simulink model "MSFartoystyring"  (R2017a)
settings: Solver=ode45  StartTime=tstart  StopTime=tstop  RelTol=1e-3  EnableMultiTasking=on
values from neighbouring files (symbols this model uses):
  c = 0    [run.m]    (also in run_task_2_2.m = 1; run_task_2_6.m = 1; run_task_2_6_without_crab_compensation.m = 1)
  chi_i_on = 0    [run_task_2_2.m]    (also in run_task_2_6.m = 1; run_task_2_6_without_crab_compensation.m)
  psi0 = 0    [run.m]    (also in run_task_2_2.m = 0.872664625997; run_task_2_6.m = 0.872664625997; run_task_2_6_without_crab_compensation.m = 0.872664625997)
  r0 = 0    [run.m]    (also in run_task_2_2.m; run_task_2_6.m; run_task_2_6_without_crab_compensation.m)
  tsamp = 10    [run.m]    (also in run_task_2_2.m; run_task_2_6.m; run_task_2_6_without_crab_compensation.m)
  v0 = [4.9 0]'    [run.m]    (also in run_task_2_2.m = [6.63 0]'; run_task_2_6.m = [6.63 0]'; run_task_2_6_without_crab_compensation.m = [6.63 0]')
undefined symbols (not defined in the file or in its folder): msfartoystyring, WP
undefined symbols (not defined in the file): p0
libraries: dspindex x2, dspswit3 x1
settings Model: ExtModeAutoUpdateStatusClock=off  Creator=christh  LastModifiedBy=jljoberg
settings DataIOCC: LimitDataPoints=on  SaveFormat=Array  SignalLoggingSaveFormat=ModelDataLogs
settings OptimizationCC: ExpressionDepthLimit=2147483647  InitFltsAndDblsToZero=on  LifeSpan=inf
settings DebuggingCC: UnderspecifiedInitializationDetection=Classic  MergeDetectMultiDrivingBlocksExec=none  SolverPrmCheckMsg=warning  StateNameClashWarn=warning  SFUnexpectedBacktrackingDiag=warning  SFNoUnconditionalDefaultTransitionDiag=warning  SFExecutionAtInitializationDiag=none
settings HardwareCC: ProdBitPerPointer=32  ProdBitPerSizeT=32  ProdBitPerPtrDiffT=32  ProdLargestAtomicFloat=None  ProdIntDivRoundTo=Undefined  ProdEndianess=Unspecified  ProdWordSize=32  ProdHWDeviceType=32-bit Generic
settings ModelReferenceCC: PropagateSignalLabelsOutOfModel=off
settings GRTTargetCC: TargetLangStandard=C89/C90 (ANSI)  GeneratePreprocessorConditionals=Disable all  CombineOutputUpdateFcns=off  GRTInterface=on
settings ConfigComp: CovMetricSettings=dw  CovHtmlReporting=on  CovSaveCumulativeToWorkspaceVar=on  CovSaveSingleToWorkspaceVar=on  CovExternalEMLEnable=off

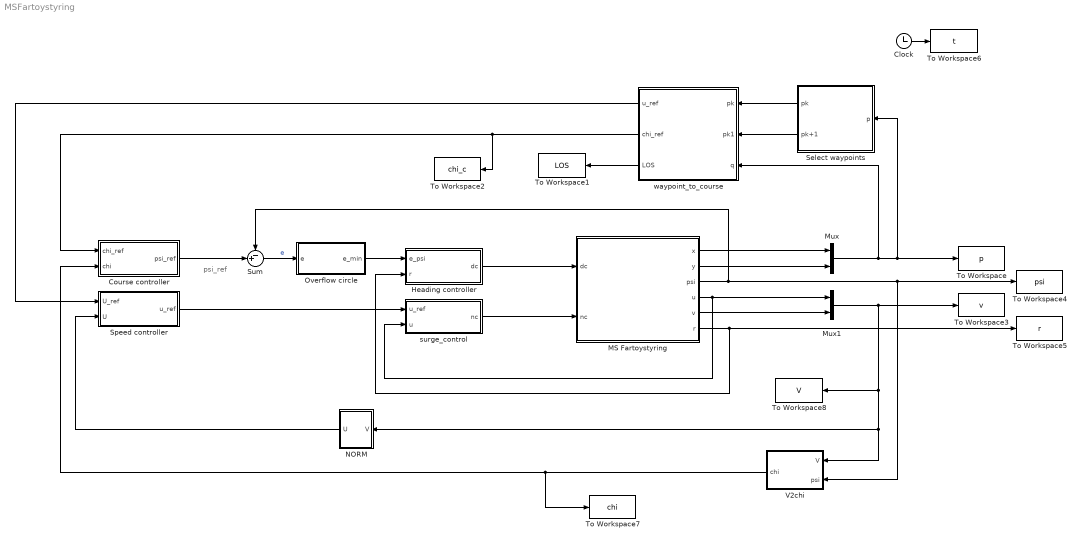
== system MSFartoystyring ==
  note: psi_ref
  Clock : Clock
  Course controller : Subsystem
  Heading controller : Subsystem
  MS Fartoystyring : Subsystem  mask(MS Fartoystyring for Assignment 3 G&C){x0=p0(1), y0=p0(2), u0=v0(1), v0=v0(2), psi0=psi0, r0=r0, c=c}
      mask prompts: x0 "x(t0) (m)"; y0 "y(t0) (m)"; u0 "u(t0) (m/s)"; v0 "v(t0) (m/s)"; psi0 "psi(t0) (rad)"; r0 "r(t0) (rad/s)"; c "current (0 or 1)"
      mask help:
      | Block corresponding to Figure 1 in the assignment text. Gives the response of the ship.
      |
      | The design speed of MS Fartoystyring is u=8.23 m/s.
      |
      | Input:
      | dc: commanded rudder (rad), dmax=25*pi/180
      | nc: commanded shaft speed (rad/s), nmax=85*2*pi/60
      |
      | Output:
      | x: north pos (m)
      | y: east pos (m)
      | u: surge (m/s)
      | v: sway (m/s)
      | psi: heading (rad)
      | r: yaw (rad/s)
      mask Help: Comments, bugs and help requests can be directed to the TA. Email on course website.
  Mux : Mux  Inputs=2
  Mux1 : Mux  Inputs=2
  NORM : MATLAB Function  TreatAsAtomicUnit=on
  Overflow circle : MATLAB Function  TreatAsAtomicUnit=on
  Select waypoints : Subsystem
  Speed controller : Subsystem
  Sum : Sum  Inputs=-+|
  To Workspace : ToWorkspace  VariableName=p  SampleTime=tsamp
  To Workspace1 : ToWorkspace  VariableName=LOS  SampleTime=tsamp
  To Workspace2 : ToWorkspace  VariableName=chi_c  SampleTime=tsamp
  To Workspace3 : ToWorkspace  VariableName=v  SampleTime=tsamp
  To Workspace4 : ToWorkspace  VariableName=psi  SampleTime=tsamp
  To Workspace5 : ToWorkspace  VariableName=r  SampleTime=tsamp
  To Workspace6 : ToWorkspace  VariableName=t  SampleTime=tsamp
  To Workspace7 : ToWorkspace  VariableName=chi  SampleTime=tsamp
  To Workspace8 : ToWorkspace  VariableName=V  SampleTime=tsamp
  V2chi : MATLAB Function  TreatAsAtomicUnit=on
  surge_control : Subsystem
  waypoint_to_course : MATLAB Function  TreatAsAtomicUnit=on
  wires:
  Clock/1 -> To Workspace6/1
  MS Fartoystyring/1(x) -> Mux/1
  MS Fartoystyring/2(y) -> Mux/2
  MS Fartoystyring/4(u) -> Mux1/1, surge_control/2(u)
  MS Fartoystyring/5(v) -> Mux1/2
  Mux1/1 -> To Workspace8/1, NORM/1(V), V2chi/1(V), To Workspace3/1
  MS Fartoystyring/6(r) -> Heading controller/2(r), To Workspace5/1
  waypoint_to_course/2(chi_ref) -> To Workspace2/1, Course controller/1(chi_ref)
  Select waypoints/1(pk) -> waypoint_to_course/1(pk)
  Select waypoints/2(pk+1) -> waypoint_to_course/2(pk1)
  Mux/1 -> To Workspace/1, Select waypoints/1(p), waypoint_to_course/3(q)
  waypoint_to_course/3(LOS) -> To Workspace1/1
  MS Fartoystyring/3(psi) -> Sum/1, To Workspace4/1, V2chi/2(psi)
  Sum/1 -> Overflow circle/1(e)  "e"
  Course controller/1(psi_ref) -> Sum/2
  surge_control/1(nc) -> MS Fartoystyring/2(nc)
  Overflow circle/1(e_min) -> Heading controller/1(e_psi)
  V2chi/1(chi) -> To Workspace7/1, Course controller/2(chi)
  Heading controller/1(dc) -> MS Fartoystyring/1(dc)
  waypoint_to_course/1(u_ref) -> Speed controller/1(U_ref)
  Speed controller/1(u_ref) -> surge_control/1(u_ref)
  NORM/1(U) -> Speed controller/2(U)

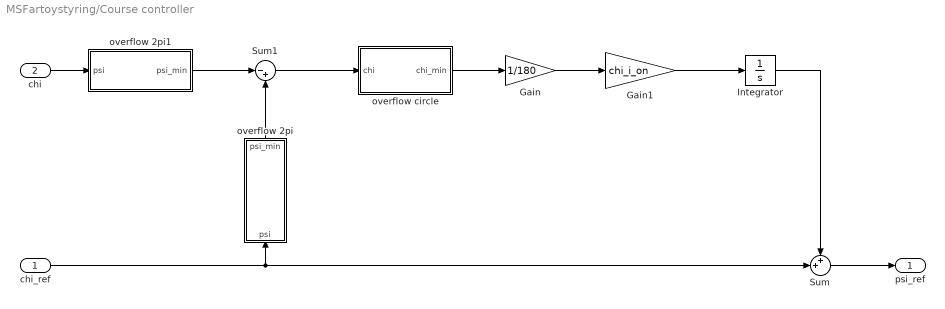
== system MSFartoystyring/Course controller ==
  chi_ref : Inport
  chi : Inport  Port=2
  Gain : Gain  Gain=1/180
  Gain1 : Gain  Gain=chi_i_on
  Integrator : Integrator  LimitOutput=on  UpperSaturationLimit=40*pi/180  LowerSaturationLimit=-40*pi/180
  Sum : Sum  Inputs=++|
  Sum1 : Sum  Inputs=|-+
  overflow 2pi : MATLAB Function  TreatAsAtomicUnit=on
  overflow 2pi1 : MATLAB Function  TreatAsAtomicUnit=on
  overflow circle : MATLAB Function  TreatAsAtomicUnit=on
  psi_ref : Outport
  wires:
  Sum/1 -> psi_ref/1
  Gain/1 -> Gain1/1
  Sum1/1 -> overflow circle/1(chi)
  chi/1 -> overflow 2pi1/1(psi)
  Integrator/1 -> Sum/1
  overflow circle/1(chi_min) -> Gain/1
  chi_ref/1 -> overflow 2pi/1(psi), Sum/2
  overflow 2pi1/1(psi_min) -> Sum1/1
  overflow 2pi/1(psi_min) -> Sum1/2
  Gain1/1 -> Integrator/1

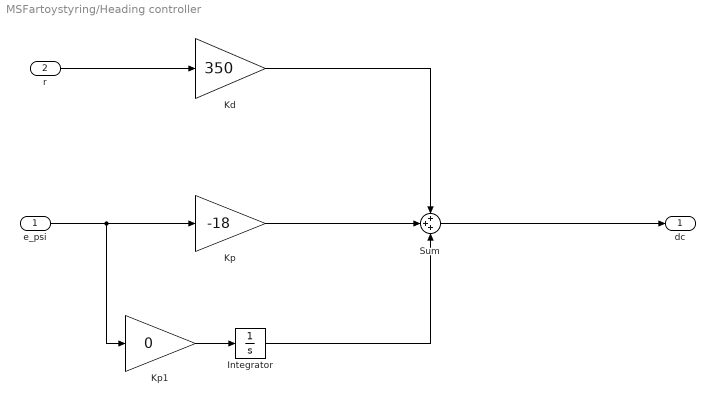
== system MSFartoystyring/Heading controller ==
  e_psi : Inport
  r : Inport  Port=2
  Integrator : Integrator
  Kd : Gain  Gain=350
  Kp : Gain  Gain=-18
  Kp1 : Gain  Gain=0
  Sum : Sum  Inputs=+++
  dc : Outport
  wires:
  e_psi/1 -> Kp1/1, Kp/1
  Sum/1 -> dc/1
  Kp/1 -> Sum/2
  r/1 -> Kd/1
  Kd/1 -> Sum/1
  Kp1/1 -> Integrator/1
  Integrator/1 -> Sum/3

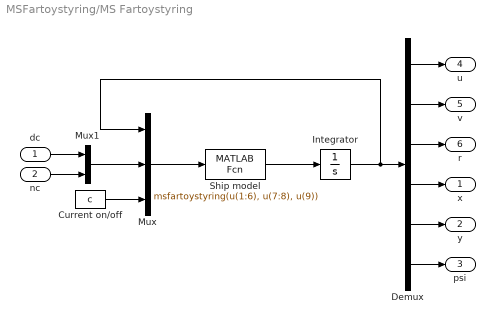
== system MSFartoystyring/MS Fartoystyring ==
  dc : Inport
  nc : Inport  Port=2
  Current on/off : Constant  Value=c
  Demux : Demux  Outputs=6
  Integrator : Integrator  InitialCondition=[u0 v0 r0 x0 y0 psi0]'
  Mux : Mux  Inputs=3
  Mux1 : Mux  Inputs=2
  Ship model : MATLABFcn  MATLABFcn=msfartoystyring(u(1:6), u(7:8), u(9))  OutputDimensions=6
  x : Outport
  y : Outport  Port=2
  psi : Outport  Port=3
  u : Outport  Port=4
  v : Outport  Port=5
  r : Outport  Port=6
  wires:
  Integrator/1 -> Mux/1, Demux/1
  Mux1/1 -> Mux/2
  dc/1 -> Mux1/1
  nc/1 -> Mux1/2
  Demux/1 -> u/1
  Demux/2 -> v/1
  Demux/3 -> r/1
  Demux/4 -> x/1
  Demux/5 -> y/1
  Demux/6 -> psi/1
  Current on/off/1 -> Mux/3
  Ship model/1 -> Integrator/1
  Mux/1 -> Ship model/1

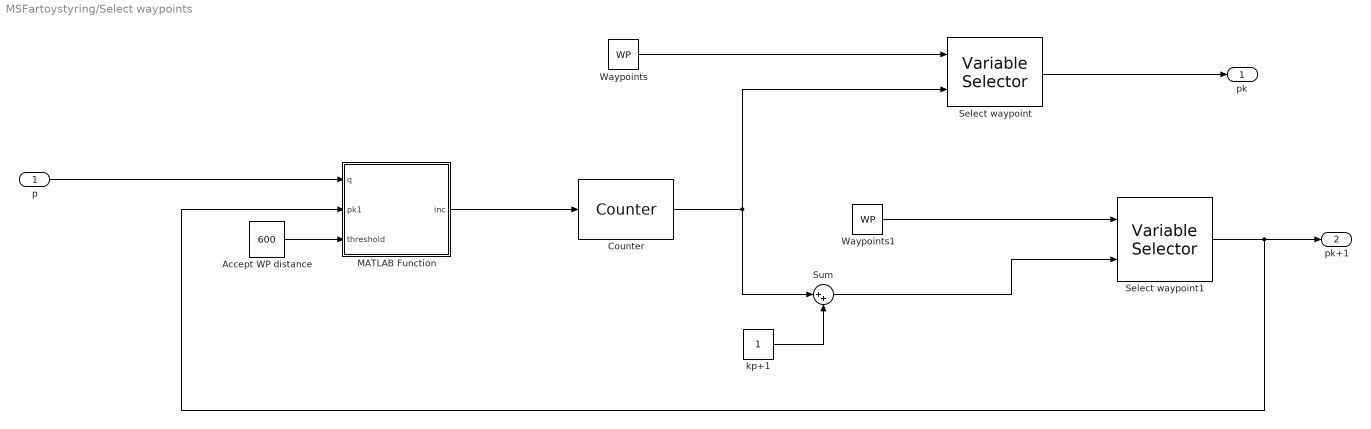
== system MSFartoystyring/Select waypoints ==
  p : Inport
  Accept WP distance : Constant  Value=600
  Counter : dspswit3/Counter  Direction=Up  CountEvent=Rising edge  CounterSize=User defined  MaxCount=7  InitialCount=0  Output=Count  HitValue=32  ResetInput=off  SamplesPerFrame=1  Ts=1  CntDtype=double  HitDtype=Logical
  MATLAB Function : MATLAB Function  TreatAsAtomicUnit=on
  Select waypoint : dspindex/Variable Selector  NumInputs=1  rowsOrCols=Columns  IdxMode=Variable  Elements=[1 3]  ZerOneIdxMode=Zero-based  errmode=Clip Index  FillMode=on  FillValues=0
  Select waypoint1 : dspindex/Variable Selector  NumInputs=1  rowsOrCols=Columns  IdxMode=Variable  Elements=[1 3]  ZerOneIdxMode=Zero-based  errmode=Clip Index  FillMode=on  FillValues=0
  Sum : Sum  Inputs=|++
  Waypoints : Constant  Value=WP
  Waypoints1 : Constant  Value=WP
  kp+1 : Constant
  pk : Outport
  pk+1 : Outport  Port=2
  wires:
  Select waypoint/1 -> pk/1
  Waypoints/1 -> Select waypoint/1
  Waypoints1/1 -> Select waypoint1/1
  Select waypoint1/1 -> MATLAB Function/2(pk1), pk+1/1
  Accept WP distance/1 -> MATLAB Function/3(threshold)
  kp+1/1 -> Sum/2
  p/1 -> MATLAB Function/1(q)
  MATLAB Function/1(inc) -> Counter/1
  Counter/1 -> Select waypoint/2, Sum/1
  Sum/1 -> Select waypoint1/2

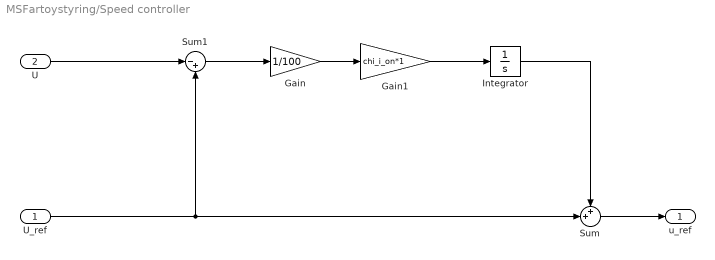
== system MSFartoystyring/Speed controller ==
  U_ref : Inport
  U : Inport  Port=2
  Gain : Gain  Gain=1/100
  Gain1 : Gain  Gain=chi_i_on*1
  Integrator : Integrator  LimitOutput=on  UpperSaturationLimit=0.3  LowerSaturationLimit=-0.3
  Sum : Sum  Inputs=++|
  Sum1 : Sum  Inputs=|-+
  u_ref : Outport
  wires:
  Sum/1 -> u_ref/1
  U/1 -> Sum1/1
  U_ref/1 -> Sum/2, Sum1/2
  Sum1/1 -> Gain/1
  Gain/1 -> Gain1/1
  Gain1/1 -> Integrator/1
  Integrator/1 -> Sum/1

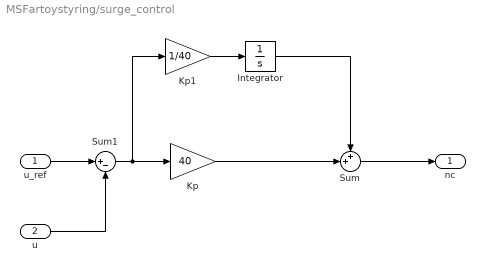
== system MSFartoystyring/surge_control ==
  u_ref : Inport
  u : Inport  Port=2
  Integrator : Integrator  LimitOutput=on  UpperSaturationLimit=8  LowerSaturationLimit=-8
  Kp : Gain  Gain=40
  Kp1 : Gain  Gain=1/40
  Sum : Sum  Inputs=++|
  Sum1 : Sum  Inputs=|+-
  nc : Outport
  wires:
  Sum/1 -> nc/1
  Kp/1 -> Sum/2
  Kp1/1 -> Integrator/1
  Integrator/1 -> Sum/1
  u/1 -> Sum1/2
  Sum1/1 -> Kp1/1, Kp/1
  u_ref/1 -> Sum1/1

== matlab function MSFartoystyring/Select waypoints/MATLAB Function ==
  data: q input; inc output; pk1 input; threshold input
function inc = fcn(q, pk1, threshold)

if norm(q-pk1)<threshold
    inc = 1;
else
    inc = 0;
end

== matlab function MSFartoystyring/waypoint_to_course ==
  data: pk input; pk1 input; q input; u_ref output; chi_ref output; LOS output
function [u_ref, chi_ref, LOS]= fcn(pk, pk1, q)

pointOnLine = @(s, pk, pk1) pk + (s)*(pk1-pk); 

persistent u_prev;
if isempty(u_prev)
    u_prev = 5;
end


% ====== Binary search to find closest point on line ========
s0 = 1/2;
delta = 1/4;
threshold = 1;          
diff = 15*threshold;
i = 0;

sA = s0; sB = s0;
while diff > threshold
    sA = s0 + delta;
    sB = s0 - delta;
    dA = norm(q - pointOnLine(sA,pk,pk1) );
    dB = norm(q - pointOnLine(sB,pk,pk1) );
    if dA < dB
        s0 = sA;
    else
        s0 = sB;
    end
    
    diff = norm(pk-pk1)*abs(sA - sB);
    delta = delta/2;
    i = i+1;
end
s = (sA+sB)/2;
% ==== Found closest point on line at <s> ========================

LAD = 600;      % Lookahead distance 
LOS = pointOnLine(s + LAD/norm(pk1-pk), pk, pk1); % Point on line to aim at


aim = LOS - q;                      % vector from boat to LOS
chi_ref = atan2(aim(2), aim(1));        % angle of aim


u_ref = min([5, u_prev+0.02]);
if norm(q-pk1) < 2*LAD
    u_ref = 3;
end

u_prev = u_ref;

== matlab function MSFartoystyring/Overflow circle ==
  data: e input; e_min output
function e_min = overflow(e)
e = mod(e,2*pi);
e_min = e;
if e > pi
    e_min = e-2*pi;
end
if e < -pi
    e_min = e+2*pi;
end

== matlab function MSFartoystyring/V2chi ==
  data: V input; chi output; psi input
function chi = V2chi(V, psi)
Rz = [cos(psi), -sin(psi); sin(psi), cos(psi)]; % BODY to NE(D) rotation

p_dot = Rz*V;
chi = atan2(p_dot(2), p_dot(1));

== matlab function MSFartoystyring/Course controller/overflow circle ==
  data: chi input; chi_min output
function chi_min = overflow(chi)
chi = mod(chi, 2*pi);
chi_min = chi;
if chi > pi
    chi_min = chi-2*pi;
end
if chi < -pi
    chi_min = chi+2*pi;
end

== matlab function MSFartoystyring/Course controller/overflow 2pi ==
  data: psi input; psi_min output
function psi_min =  oTo2pi(psi)
psi_min = mod(psi,2*pi);

== matlab function MSFartoystyring/Course controller/overflow 2pi1 ==
  data: psi input; psi_min output
function psi_min =  oTo2pi(psi)
psi_min = mod(psi,2*pi);

== matlab function MSFartoystyring/NORM ==
  data: V input; U output
function U = norm(V)
U = norm(V);
